simulink model "crtb_model"  (R2021b)
settings: Solver=FixedStepAuto  StartTime=0.0  StopTime=1  FixedStep=0.01  RelTol=1e-3
values from neighbouring files (symbols this model uses):
  A = [0 1 0 0; -K/M 0 K/M 0; 0 0 0 1; K/M 0 -K/M 0]    [desafio1.m]
  B = [0 0; 1/M 0; 0 0; 0 1/M]    [desafio1.m]
  C = eye(4)    [desafio1.m]
  D = [0 0; 0 0;0 0;0 0]    [desafio1.m]
  x0 = [0; 0; 0; 0]    [desafio1.m]
settings Model: Creator=Murillo  LastModifiedBy=Murillo

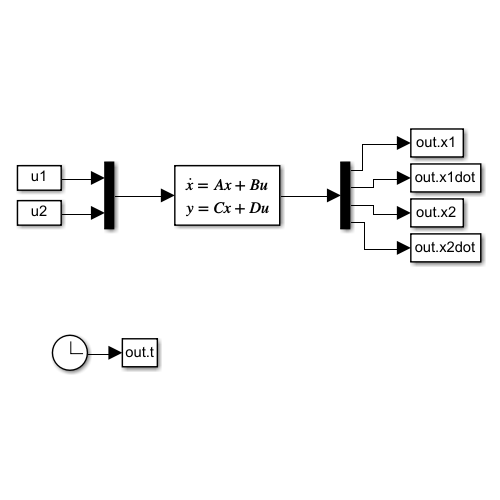
[thumbnail: Simulink's stored preview of the top-level diagram]
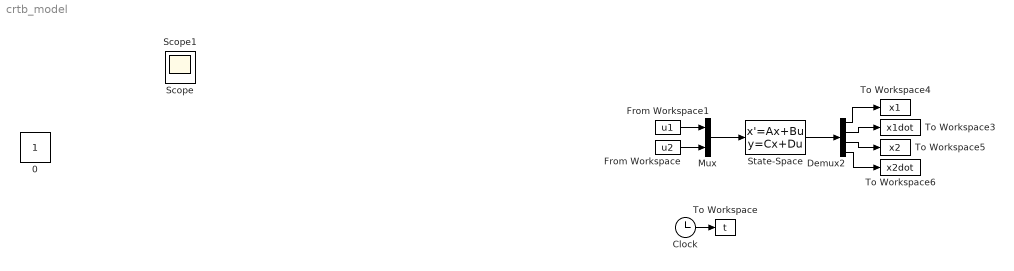
== system crtb_model ==
  Clock : Clock
  Demux2 : Demux
  From Workspace : FromWorkspace  VariableName=u2
  From Workspace1 : FromWorkspace  VariableName=u1
  Mux : Mux  Inputs=2
  State-Space : StateSpace  A=A  B=B  C=C  D=D  InitialCondition=x0
  To Workspace : ToWorkspace  VariableName=t  SampleTime=-1
      settings: Save2DSignal=2-D array (concatenate along first dimension)
  To Workspace3 : ToWorkspace  VariableName=x1dot  SampleTime=-1
      settings: Save2DSignal=2-D array (concatenate along first dimension)
  To Workspace4 : ToWorkspace  VariableName=x1  SampleTime=-1
      settings: Save2DSignal=2-D array (concatenate along first dimension)
  To Workspace5 : ToWorkspace  VariableName=x2  SampleTime=-1
      settings: Save2DSignal=2-D array (concatenate along first dimension)
  To Workspace6 : ToWorkspace  VariableName=x2dot  SampleTime=-1
      settings: Save2DSignal=2-D array (concatenate along first dimension)
  0 : Constant  IOType=siggen
  Scope : Scope
  Scope1 : Scope
  wires:
  Clock/1 -> To Workspace/1
  State-Space/1 -> Demux2/1
  Demux2/1 -> To Workspace4/1
  Demux2/4 -> To Workspace6/1
  Demux2/3 -> To Workspace5/1
  Demux2/2 -> To Workspace3/1
  From Workspace1/1 -> Mux/1
  From Workspace/1 -> Mux/2
  Mux/1 -> State-Space/1
